simulink model "Simulacion_Completa_DET_M1"  (R2023a)
settings: Solver=VariableStepAuto  StartTime=0.0  StopTime=6062  RelTol=1e-3
undefined symbols (not defined in the file): Ion, Lithium
libraries: spsSeriesRLCBranchLib x15, spsIdealSwitchLib x11, slpidlib x3, spsCurrentMeasurementLib x2, spsIGBTDiodeLib x2, SignalEditorBlockLib x2, spsVoltageMeasurementLib x2, spsBatteryLib x1, spsBoostConverterLib x1, simulink x1, spsDiodeLib x1, eeGeneralControl x1
settings Model: SimulationMode=accelerator  Creator=javie  LastModifiedBy=javie
settings DebuggingCC: ParameterPrecisionLossMsg=none

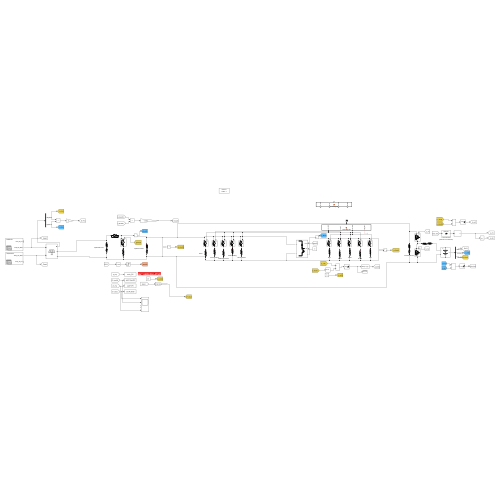
[thumbnail: Simulink's stored preview of the top-level diagram]
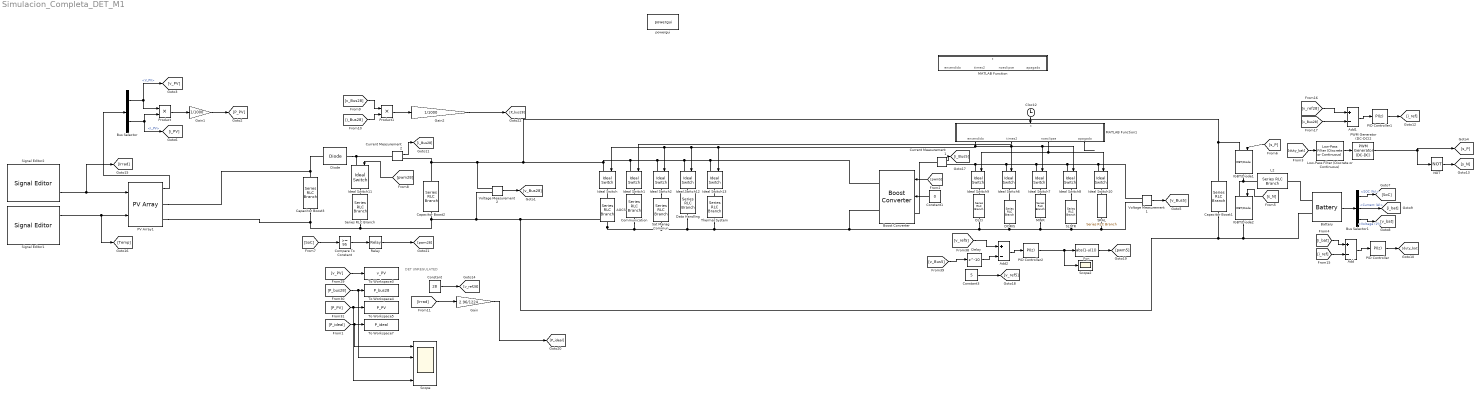
== system Simulacion_Completa_DET_M1 ==
  note: DET UNREGULATED
  AOCS : spsSeriesRLCBranchLib/Series RLC Branch  LConnTagsString=__new0  RConnTagsString=__new0  BranchType=R  Resistance=6.53  Inductance=1e-3  SetiL0=off  InitialCurrent=0  Capacitance=3300e-6  Setx0=off  InitialVoltage=0  Measurements=None
  Add : Sum  Inputs=+-
  Add1 : Sum  Inputs=+-
  Add2 : Sum  Inputs=+-
  Battery : spsBatteryLib/Battery  BatType=Lithium-Ion  ShowTempParam=off  ThermalPreset=no  ShowAgeParam=off  NomV=26  NomQ=60  SOC=60  Batt_Tr=1  PresetModel=on  MaxQ=60  MinV=19.5  FullV=30.2637  Dis_rate=26.087  R=0.0043333  Normal_OP=54.2609  expZone="[28.09      2.94783]"  current=[6.5 13 32.5]  Units=Time  Tci=20  NomT=20  T2=-30  MaxQ2=4.8  FullV2=7.1  Normal_OP2=5.655  expZone2="[6.58           1]"  Rca=0.6  ti=2000  Dp=0  Neq0=0  Tsim=1e6  Ta1=25  Qeol=5.4*0.9  Reol=0.013333*1.2  Char_age=[2.3478, 3]  Dis_age=[2.3478, 10]  N1=1500  N2=10500  N3=1000  N4=1400  Ta2=45  N5=950
  Boost Converter : spsBoostConverterLib/Boost Converter  ModelType=Average model (No rectifier mode)  Ron=1e-3  Rs=1e6  Cs=inf  Vforward=[0,0]  Ron_Diode=1e-3  Rs_Diode=1e6  Cs_Diode=inf  Vf_Diode=1e-3  Rs_CurrentSource=inf  Ron_ACsource=1e-3
      settings: LibrarySourceBlock=sps_lib/Power Electronics/Boost Converter
  Bus Selector : BusSelector  OutputSignals=V_PV,I_PV
  Bus Selector1 : BusSelector  OutputSignals=SOC (%),Current (A),Voltage (V)
  Capacitor Boost1 : spsSeriesRLCBranchLib/Series RLC Branch  LConnTagsString=__new0  RConnTagsString=__new0  BranchType=RC  Resistance=1e-4  Inductance=1e-3  SetiL0=off  InitialCurrent=0  Capacitance=1000e-6  Setx0=off  InitialVoltage=0  Measurements=None
  Capacitor Boost2 : spsSeriesRLCBranchLib/Series RLC Branch  LConnTagsString=__new0  RConnTagsString=__new0  BranchType=RC  Resistance=1e-4  Inductance=1e-3  SetiL0=off  InitialCurrent=0  Capacitance=1000e-6  Setx0=off  InitialVoltage=0  Measurements=None
  Capacitor Boost3 : spsSeriesRLCBranchLib/Series RLC Branch  LConnTagsString=__new0  RConnTagsString=__new0  BranchType=RC  Resistance=1e-4  Inductance=1e-3  SetiL0=off  InitialCurrent=0  Capacitance=1000e-6  Setx0=off  InitialVoltage=0  Measurements=None
  Clock2 : Clock
  Communication : spsSeriesRLCBranchLib/Series RLC Branch  LConnTagsString=__new0  RConnTagsString=__new0  BranchType=R  Resistance=5.23  Inductance=1e-3  SetiL0=off  InitialCurrent=0  Capacitance=3300e-6  Setx0=off  InitialVoltage=0  Measurements=None
  Compare To Constant : simulink/Logic and Bit Operations/Compare To Constant  relop=>=  const=95  OutDataTypeStr=boolean
  Constant : Constant  Value=28
  Constant1 : Constant  Value=0
  Constant3 : Constant  Value=5
  Current Measurement1 : spsCurrentMeasurementLib/Current Measurement  PhasorSimulation=off  OutputType=Complex  PSBequivalent=0
  Current Measurement2 : spsCurrentMeasurementLib/Current Measurement  PhasorSimulation=off  OutputType=Complex  PSBequivalent=0
  DORIS : spsSeriesRLCBranchLib/Series RLC Branch  LConnTagsString=__new0  RConnTagsString=__new0  BranchType=R  Resistance=1  Inductance=1e-3  SetiL0=off  InitialCurrent=0  Capacitance=3300e-6  Setx0=off  InitialVoltage=0  Measurements=None
  Data Handling : spsSeriesRLCBranchLib/Series RLC Branch  LConnTagsString=__new0  RConnTagsString=__new0  BranchType=R  Resistance=7.84  Inductance=1e-3  SetiL0=off  InitialCurrent=0  Capacitance=3300e-6  Setx0=off  InitialVoltage=0  Measurements=None
  Delay : Delay  DelayLength=10
  Diode : spsDiodeLib/Diode  Ron=0.001  Lon=0  Vf=0.8  IC=0  UseSnubber=0  Rs=500  Cs=250e-9  Measurements=off
  Fcn : Fcn  Expr=abs(1-u(1))
  Gain : Gain  Gain=2.96/1224  OutDataTypeStr=Inherit: Same as input
  Gain1 : Gain  Gain=1/1000
  Gain2 : Gain  Gain=1/1000
  IGBT/Diode1 : spsIGBTDiodeLib/IGBT//Diode  Ron=1e-3  Rs=1e5  Cs=inf  Measurements=off
  IGBT/Diode2 : spsIGBTDiodeLib/IGBT//Diode  Ron=1e-3  Rs=1e5  Cs=inf  Measurements=off
  Ideal Switch{,1..2,6..13} (11 alike) : spsIdealSwitchLib/Ideal Switch  Ron=0.001  Lon=0  IC=0  Rs=1e5  Cs=inf  Measurements=off
  L2 : spsSeriesRLCBranchLib/Series RLC Branch  LConnTagsString=__new0  RConnTagsString=__new0  BranchType=RL  Resistance=0.1  Inductance=0.5e-3  SetiL0=off  InitialCurrent=0  Capacitance=1e-6  Setx0=off  InitialVoltage=0  Measurements=None
  Low-Pass Filter (Discrete or Continuous) : eeGeneralControl/Low-Pass Filter (Discrete or Continuous)  K=1  T=1  B=inf  A=-inf  init_option=Inherited from block input  x0=0  Ts=-1
  MATLAB Function : MATLAB Function  TreatAsAtomicUnit=on
  MATLAB Function1 : MATLAB Function  TreatAsAtomicUnit=on
  MWR : spsSeriesRLCBranchLib/Series RLC Branch  LConnTagsString=__new0  RConnTagsString=__new0  BranchType=R  Resistance=0.74  Inductance=1e-3  SetiL0=off  InitialCurrent=0  Capacitance=3300e-6  Setx0=off  InitialVoltage=0  Measurements=None
  NOT : Logic  Operator=NOT  AllPortsSameDT=off  OutDataTypeStr=boolean
  OLCI : spsSeriesRLCBranchLib/Series RLC Branch  LConnTagsString=__new0  RConnTagsString=__new0  BranchType=R  Resistance=0.2  Inductance=1e-3  SetiL0=off  InitialCurrent=0  Capacitance=3300e-6  Setx0=off  InitialVoltage=0  Measurements=None
  PID Controller : slpidlib/PID Controller  Controller=PI  Form=Parallel  TimeDomain=Discrete-time  UseExternalTs=off  SampleTime=50e-6  IntegratorMethod=Forward Euler  FilterMethod=Forward Euler  ControllerParametersSource=internal  P=0.8  I=10  UseKiTs=off  D=0  N=100  UseFilter=on  TunerSelectOption=Frequency Response Based  InitialConditionSource=internal  InitialConditionForIntegrator=0  InitialConditionForFilter=0  DifferentiatorICPrevScaledInput=0  ExternalReset=none  TrackingMode=off  Kt=1  LimitOutput=on  SatLimitsSource=internal  UpperSaturationLimit=0.95  LowerSaturationLimit=0  LinearizeAsGain=on  AntiWindupMode=none  Kb=1  LimitIntegrator=off  UpperIntegratorSaturationLimit=inf  LowerIntegratorSaturationLimit=-inf  POutMin=[]  POutMax=[]  IOutMin=[]  IOutMax=[]  DOutMin=[]  DOutMax=[]  NOutMin=[]  NOutMax=[]  SumOutMin=[]  SumOutMax=[]  SaturationOutMin=[]  SaturationOutMax=[]  PParamMin=[]  PParamMax=[]  IParamMin=[]  IParamMax=[]  DParamMin=[]  DParamMax=[]  NParamMin=[]  NParamMax=[]  KbParamMin=[]  KbParamMax=[]  KtParamMin=[]  KtParamMax=[]  KbOutMin=[]  KbOutMax=[]  KtOutMin=[]  KtOutMax=[]  IntegratorOutMin=[]  IntegratorOutMax=[]  FilterOutMin=[]  FilterOutMax=[]  SumI1OutMin=[]  SumI1OutMax=[]  SumI2OutMin=[]  SumI2OutMax=[]  SumI3OutMin=[]  SumI3OutMax=[]  SumI4OutMin=[]  SumI4OutMax=[]  SumDOutMin=[]  SumDOutMax=[]  DifferentiatorOutMin=[]  DifferentiatorOutMax=[]  FilterDiffOutCoefMin=[]  FilterDiffOutCoefMax=[]  ReciprocalOutMin=[]  ReciprocalOutMax=[]  SumDenOutMin=[]  SumDenOutMax=[]  SumNumOutMin=[]  SumNumOutMax=[]  DivideOutMin=[]  DivideOutMax=[]  UdiffTsProdOutMin=[]  UdiffTsProdOutMax=[]  NTsProdOutMin=[]  NTsProdOutMax=[]  UintegralTsProdOutMin=[]  UintegralTsProdOutMax=[]  UngainTsProdOutMin=[]  UngainTsProdOutMax=[]  ClampingZeroOutDataTypeStr=Inherit: Inherit via back propagation  ClampingZeroOutMin=[]  ClampingZeroOutMax=[]  FilterDenConstantOutDataTypeStr=Inherit: Inherit via back propagation  FilterDenConstantOutMin=[]  FilterDenConstantOutMax=[]  PCopyOutDataTypeStr=Inherit: Inherit via back propagation  PCopyOutMin=[]  PCopyOutMax=[]  NCopyOutDataTypeStr=Inherit: Inherit via back propagation  NCopyOutMin=[]  NCopyOutMax=[]  IntegratorContinuousStateAttributes=''  IntegratorStateMustResolveToSignalObject=off  IntegratorRTWStateStorageClass=Auto  FilterContinuousStateAttributes=''  FilterStateMustResolveToSignalObject=off  FilterRTWStateStorageClass=Auto  ParallelPVariant=InternalParameters  IdealPVariant=Disabled  IVariant=InternalParameters  DVariant=Disabled  IntegratorVariant=Discrete  SatVariant=Enabled  AWVariant=Passthrough  PCopyVariant=Disabled  TRVariant=Disabled  FdbkBlocksVariant=Forward  IdealPFdbkVariant=Disabled  SatFdbkVariant=Disabled  DerivativeFilterVariant=Disabled  NVariant=Disabled  NCopyVariant=Disabled_SignalSpec  FilterICVariant=Disabled  IntegratorICVariant=InternalICs  ExternalResetVariant=Disabled  TRSumVariant=Passthrough  SumFdbkVariant=Disabled  SumVariant=Sum_PI  TsampFilterVariant=InternalTs  TsampNgainVariant=Passthrough  TsampIntegralVariant=Disabled_SignalSpec  ExternalSaturationOutDataTypeStr=Inherit: Same as second input
  PID Controller1 : slpidlib/PID Controller  Controller=PI  Form=Parallel  TimeDomain=Discrete-time  UseExternalTs=off  SampleTime=500e-6  IntegratorMethod=Forward Euler  FilterMethod=Forward Euler  ControllerParametersSource=internal  P=0.85  I=10  UseKiTs=off  D=0  N=100  UseFilter=on  TunerSelectOption=Transfer Function Based (PID Tuner App)  InitialConditionSource=internal  InitialConditionForIntegrator=0  InitialConditionForFilter=0  DifferentiatorICPrevScaledInput=0  ExternalReset=none  TrackingMode=off  Kt=1  LimitOutput=on  SatLimitsSource=internal  UpperSaturationLimit=40  LowerSaturationLimit=-40  LinearizeAsGain=on  AntiWindupMode=none  Kb=1  LimitIntegrator=off  UpperIntegratorSaturationLimit=inf  LowerIntegratorSaturationLimit=-inf  RndMeth=Zero  POutMin=[]  POutMax=[]  IOutMin=[]  IOutMax=[]  DOutMin=[]  DOutMax=[]  NOutMin=[]  NOutMax=[]  SumOutMin=[]  SumOutMax=[]  SaturationOutMin=[]  SaturationOutMax=[]  PParamMin=[]  PParamMax=[]  IParamMin=[]  IParamMax=[]  DParamMin=[]  DParamMax=[]  NParamMin=[]  NParamMax=[]  KbParamMin=[]  KbParamMax=[]  KtParamMin=[]  KtParamMax=[]  KbOutMin=[]  KbOutMax=[]  KtOutMin=[]  KtOutMax=[]  IntegratorOutMin=[]  IntegratorOutMax=[]  FilterOutMin=[]  FilterOutMax=[]  SumI1OutMin=[]  SumI1OutMax=[]  SumI2OutMin=[]  SumI2OutMax=[]  SumI3OutMin=[]  SumI3OutMax=[]  SumI4OutMin=[]  SumI4OutMax=[]  SumDOutMin=[]  SumDOutMax=[]  DifferentiatorOutMin=[]  DifferentiatorOutMax=[]  FilterDiffOutCoefMin=[]  FilterDiffOutCoefMax=[]  ReciprocalOutMin=[]  ReciprocalOutMax=[]  SumDenOutMin=[]  SumDenOutMax=[]  SumNumOutMin=[]  SumNumOutMax=[]  DivideOutMin=[]  DivideOutMax=[]  UdiffTsProdOutMin=[]  UdiffTsProdOutMax=[]  NTsProdOutMin=[]  NTsProdOutMax=[]  UintegralTsProdOutMin=[]  UintegralTsProdOutMax=[]  UngainTsProdOutMin=[]  UngainTsProdOutMax=[]  ClampingZeroOutDataTypeStr=Inherit: Inherit via back propagation  ClampingZeroOutMin=[]  ClampingZeroOutMax=[]  FilterDenConstantOutDataTypeStr=Inherit: Inherit via back propagation  FilterDenConstantOutMin=[]  FilterDenConstantOutMax=[]  PCopyOutDataTypeStr=Inherit: Inherit via back propagation  PCopyOutMin=[]  PCopyOutMax=[]  NCopyOutDataTypeStr=Inherit: Inherit via back propagation  NCopyOutMin=[]  NCopyOutMax=[]  IntegratorContinuousStateAttributes=''  IntegratorStateMustResolveToSignalObject=off  IntegratorRTWStateStorageClass=Auto  FilterContinuousStateAttributes=''  FilterStateMustResolveToSignalObject=off  FilterRTWStateStorageClass=Auto  ParallelPVariant=InternalParameters  IdealPVariant=Disabled  IVariant=InternalParameters  DVariant=Disabled  IntegratorVariant=Discrete  SatVariant=Enabled  AWVariant=Passthrough  PCopyVariant=Disabled  TRVariant=Disabled  FdbkBlocksVariant=Forward  IdealPFdbkVariant=Disabled  SatFdbkVariant=Disabled  DerivativeFilterVariant=Disabled  NVariant=Disabled  NCopyVariant=Disabled_SignalSpec  FilterICVariant=Disabled  IntegratorICVariant=InternalICs  ExternalResetVariant=Disabled  TRSumVariant=Passthrough  SumFdbkVariant=Disabled  SumVariant=Sum_PI  TsampFilterVariant=InternalTs  TsampNgainVariant=Passthrough  TsampIntegralVariant=Disabled_SignalSpec  ExternalSaturationOutDataTypeStr=Inherit: Same as second input
  PID Controller2 : slpidlib/PID Controller  Controller=PI  Form=Parallel  TimeDomain=Discrete-time  UseExternalTs=off  SampleTime=50e-6  IntegratorMethod=Forward Euler  FilterMethod=Forward Euler  ControllerParametersSource=internal  P=0.02  I=1  UseKiTs=off  D=0  N=100  UseFilter=on  TunerSelectOption=Frequency Response Based  InitialConditionSource=internal  InitialConditionForIntegrator=0  InitialConditionForFilter=0  DifferentiatorICPrevScaledInput=0  ExternalReset=none  TrackingMode=off  Kt=1  LimitOutput=on  SatLimitsSource=internal  UpperSaturationLimit=0.999  LowerSaturationLimit=0  LinearizeAsGain=off  AntiWindupMode=none  Kb=1  LimitIntegrator=off  UpperIntegratorSaturationLimit=inf  LowerIntegratorSaturationLimit=-inf  POutMin=[]  POutMax=[]  IOutMin=[]  IOutMax=[]  DOutMin=[]  DOutMax=[]  NOutMin=[]  NOutMax=[]  SumOutMin=[]  SumOutMax=[]  SaturationOutMin=[]  SaturationOutMax=[]  PParamMin=[]  PParamMax=[]  IParamMin=[]  IParamMax=[]  DParamMin=[]  DParamMax=[]  NParamMin=[]  NParamMax=[]  KbParamMin=[]  KbParamMax=[]  KtParamMin=[]  KtParamMax=[]  KbOutMin=[]  KbOutMax=[]  KtOutMin=[]  KtOutMax=[]  IntegratorOutMin=[]  IntegratorOutMax=[]  FilterOutMin=[]  FilterOutMax=[]  SumI1OutMin=[]  SumI1OutMax=[]  SumI2OutMin=[]  SumI2OutMax=[]  SumI3OutMin=[]  SumI3OutMax=[]  SumI4OutMin=[]  SumI4OutMax=[]  SumDOutMin=[]  SumDOutMax=[]  DifferentiatorOutMin=[]  DifferentiatorOutMax=[]  FilterDiffOutCoefMin=[]  FilterDiffOutCoefMax=[]  ReciprocalOutMin=[]  ReciprocalOutMax=[]  SumDenOutMin=[]  SumDenOutMax=[]  SumNumOutMin=[]  SumNumOutMax=[]  DivideOutMin=[]  DivideOutMax=[]  UdiffTsProdOutMin=[]  UdiffTsProdOutMax=[]  NTsProdOutMin=[]  NTsProdOutMax=[]  UintegralTsProdOutMin=[]  UintegralTsProdOutMax=[]  UngainTsProdOutMin=[]  UngainTsProdOutMax=[]  ClampingZeroOutDataTypeStr=Inherit: Inherit via back propagation  ClampingZeroOutMin=[]  ClampingZeroOutMax=[]  FilterDenConstantOutDataTypeStr=Inherit: Inherit via back propagation  FilterDenConstantOutMin=[]  FilterDenConstantOutMax=[]  PCopyOutDataTypeStr=Inherit: Inherit via back propagation  PCopyOutMin=[]  PCopyOutMax=[]  NCopyOutDataTypeStr=Inherit: Inherit via back propagation  NCopyOutMin=[]  NCopyOutMax=[]  IntegratorContinuousStateAttributes=''  IntegratorStateMustResolveToSignalObject=off  IntegratorRTWStateStorageClass=Auto  FilterContinuousStateAttributes=''  FilterStateMustResolveToSignalObject=off  FilterRTWStateStorageClass=Auto  ParallelPVariant=InternalParameters  IdealPVariant=Disabled  IVariant=InternalParameters  DVariant=Disabled  IntegratorVariant=Discrete  SatVariant=Enabled  AWVariant=Passthrough  PCopyVariant=Disabled  TRVariant=Disabled  FdbkBlocksVariant=Forward  IdealPFdbkVariant=Disabled  SatFdbkVariant=Disabled  DerivativeFilterVariant=Disabled  NVariant=Disabled  NCopyVariant=Disabled_SignalSpec  FilterICVariant=Disabled  IntegratorICVariant=InternalICs  ExternalResetVariant=Disabled  TRSumVariant=Passthrough  SumFdbkVariant=Disabled  SumVariant=Sum_PI  TsampFilterVariant=InternalTs  TsampNgainVariant=Passthrough  TsampIntegralVariant=Disabled_SignalSpec  ExternalSaturationOutDataTypeStr=Inherit: Same as second input
  PV Array1 : spsPVArrayLib/PV Array  Npar=7  Nser=2  PlotType=array @ 25 deg.C & specified irradiances  S_vec=[ 1200 1000 800 400 ]  Temp_C_vec="[ 45 25  ]"  ModuleName=Solartech Energy ASC-6P-48-180  PlotWhenSelected=off  Pm=180.0288  Ncell=48  Voc=29.2  Isc=8.48  Vm=22.56  Im=7.98  beta_Voc_pc=-0.36  alpha_Isc_pc=0.06  beta_Voc=-0.10512  alpha_Isc=0.005088  IL=8.5066  I0=2.8822e-10  nI=0.9824  Rsh=559.0814  Rs=0.40197  RobustModel=off  RobustCellTemperature=313.3991  BAL=on  Tc=1e-6  Tfilter=5e-5
  PWM Generator (DC-DC)2 : spsPWMGeneratorDCDCLib/PWM Generator (DC-DC)  Fsw=20000  Ts=1e-4
  Product : Product
  Product1 : Product
  Relay : Relay
  SLSTR : spsSeriesRLCBranchLib/Series RLC Branch  LConnTagsString=__new0  RConnTagsString=__new0  BranchType=R  Resistance=0.16  Inductance=1e-3  SetiL0=off  InitialCurrent=0  Capacitance=3300e-6  Setx0=off  InitialVoltage=0  Measurements=None
  SRAL : spsSeriesRLCBranchLib/Series RLC Branch  LConnTagsString=__new0  RConnTagsString=__new0  BranchType=R  Resistance=0.28  Inductance=1e-3  SetiL0=off  InitialCurrent=0  Capacitance=3300e-6  Setx0=off  InitialVoltage=0  Measurements=None
  Sat Manag Commun : spsSeriesRLCBranchLib/Series RLC Branch  LConnTagsString=__new0  RConnTagsString=__new0  BranchType=R  Resistance=6.03  Inductance=1e-3  SetiL0=off  InitialCurrent=0  Capacitance=3300e-6  Setx0=off  InitialVoltage=0  Measurements=None
  Scope : Scope  NumInputPorts=4
  Scope2 : Scope
  Series RLC Branch : spsSeriesRLCBranchLib/Series RLC Branch  LConnTagsString=__new0  RConnTagsString=__new0  BranchType=R  Resistance=1  Inductance=1e-3  SetiL0=off  InitialCurrent=0  Capacitance=1e-6  Setx0=off  InitialVoltage=0  Measurements=None
  Signal Editor1 : SignalEditorBlockLib/Signal Editor  FileName=Irradiancias_signal_6062.mat  ActiveScenario=Temperatura  ActiveSignal=Temp_50_6062  IsBus=off  OutputBusObjectStr=Bus: BusObject  SampleTime=0  Interpolate=off  ZeroCross=off  OutputAfterFinalValue=Setting to zero  Unit=inherit  PreserveSignalName=on  ApplySigPropsToAllScenarios=off
  Signal Editor2 : SignalEditorBlockLib/Signal Editor  FileName=Irradiancias_signal_6062.mat  ActiveScenario=Irradiancia  ActiveSignal=Irrad_50_10  IsBus=off  OutputBusObjectStr=Bus: BusObject  SampleTime=0  Interpolate=off  ZeroCross=off  OutputAfterFinalValue=Setting to zero  Unit=inherit  PreserveSignalName=on  ApplySigPropsToAllScenarios=off
  Thermal System : spsSeriesRLCBranchLib/Series RLC Branch  LConnTagsString=__new0  RConnTagsString=__new0  BranchType=R  Resistance=9.8  Inductance=1e-3  SetiL0=off  InitialCurrent=0  Capacitance=3300e-6  Setx0=off  InitialVoltage=0  Measurements=None
  To Workspace3 : ToWorkspace  VariableName=v_PV  SaveFormat=Structure With Time  SampleTime=-1
      settings: Decimation=10000
  To Workspace4 : ToWorkspace  VariableName=P_bus28  SaveFormat=Structure With Time  SampleTime=-1
      settings: Decimation=10000
  To Workspace5 : ToWorkspace  VariableName=P_PV  SaveFormat=Structure With Time  SampleTime=-1
      settings: Decimation=10000
  To Workspace7 : ToWorkspace  VariableName=P_ideal  SaveFormat=Structure With Time  SampleTime=-1
      settings: Decimation=10000
  Voltage Measurement1 : spsVoltageMeasurementLib/Voltage Measurement  PhasorSimulation=off  OutputType=Complex  PSBequivalent=0
  Voltage Measurement2 : spsVoltageMeasurementLib/Voltage Measurement  PhasorSimulation=off  OutputType=Complex  PSBequivalent=0
  powergui : sps_lib/powergui  Priority=1  SimulationMode=Discrete  SampleTime=1e-4  frequency=60  Iterations=50  frequencyindice=0  Pbase=100e6  ErrMax=1e-4  UnitsV=kV  UnitsW=MW  buscounter=0  FunctionMessages=off  echomessages=off  EnableUseOfTLC=off  CurrentSourceSwitches=off  DisableSnubberDevices=off  DisableRonSwitches=off  DisableVfSwitches=off  DisplayEquations=off  AutomaticDiscreteSolvers=off  SolverType=Tustin/Backward Euler (TBE)  Interpol=off  ExternalGateDelay=off  methode=off  Ts=100  x0status=blocks  SPID=on  SwTol=0  HookPort=off  NonlinearTolerance=1e-4  nMaxIteration=100  ContinueOnMaxIteration=off  RestoreLinks=warning  ResistiveCurrentMeasurement=off  Frange=[0:2:500]  Ylog=off  Xlog=on  ShowGrid=off  save=off  variable=ZData  structure=0  ZoomFFT=off  StartTime=0.0  cycles=1  DisplayStyle=1  fundamental=60  FreqAxis=off  MaxFrequency=1000  frequencyindicesteady=1  RmsSteady=1  display=off
  wires:
  [pwm28] -> Ideal Switch11/1
  Relay/1 -> [pwm28]
  [SoC] -> Compare To Constant/1
  Current Measurement2/1 -> [i_Bus28]
  Compare To Constant/1 -> Relay/1
  PV Array1/1 -> Bus Selector/1
  Gain1/1 -> [P_PV]
  Bus Selector/2 -> Product/2, [i_PV]  "<I_PV>"
  Bus Selector/1 -> Product/1, [v_PV]  "<V_PV>"
  Product/1 -> Gain1/1
  [P_ideal] -> Scope/1, To Workspace7/1
  [P_bus28] -> Scope/2, To Workspace4/1
  Constant/1 -> [v_ref28]
  [Irrad] -> Gain/1
  Gain/1 -> [P_ideal]
  [v_PV] -> To Workspace3/1
  [P_PV] -> Scope/4, To Workspace5/1
  [v_Bus28] -> Add1/2
  NOT/1 -> [s_N]
  [duty_bat] -> Low-Pass Filter (Discrete or Continuous)/1
  [s_P] -> IGBT/Diode1/1
  Add1/1 -> PID Controller1/1
  [i_bat] -> Add/1
  Bus Selector1/3 -> [v_bat]  "<Voltage (V)>"
  [v_ref28] -> Add1/1
  PWM Generator (DC-DC)2/1 -> [s_P], NOT/1
  [i_ref] -> Add/2
  PID Controller/1 -> [duty_bat]
  Battery/1 -> Bus Selector1/1
  Add/1 -> PID Controller/1
  Bus Selector1/1 -> [SoC]  "<SOC (%)>"
  [s_N] -> IGBT/Diode2/1
  Bus Selector1/2 -> [i_bat]  "<Current (A)>"
  Low-Pass Filter (Discrete or Continuous)/1 -> PWM Generator (DC-DC)2/1
  PID Controller1/1 -> [i_ref]
  Constant1/1 -> Boost Converter/2
  Add2/1 -> PID Controller2/1
  Fcn/1 -> [pwm5]
  Delay/1 -> Add2/2
  Current Measurement1/1 -> [i_Bus5]
  [v_Bus5] -> Delay/1
  Voltage Measurement1/1 -> [v_Bus5]
  Constant3/1 -> [v_ref5]
  MATLAB Function1/3(noeclipse) -> Ideal Switch10/1, Ideal Switch9/1
  [v_ref5] -> Add2/1
  PID Controller2/1 -> Scope2/1, Fcn/1
  Clock2/1 -> MATLAB Function1/1(t)
  [pwm5] -> Boost Converter/1
  MATLAB Function1/4(apagado) -> ?
  MATLAB Function1/1(encendido) -> Ideal Switch8/1, Ideal Switch7/1, Ideal Switch6/1, Ideal Switch/1, Ideal Switch2/1, Ideal Switch12/1, Ideal Switch13/1
  Signal Editor2/2 -> [Irrad], PV Array1/1
  Signal Editor1/1 -> [Temp], PV Array1/2
  MATLAB Function1/2(times2) -> Ideal Switch1/1
  Voltage Measurement2/1 -> [v_Bus28]
  Product1/1 -> Gain2/1
  Gain2/1 -> [P_bus28]
  [v_Bus28] -> Product1/1
  [i_Bus28] -> Product1/2
  connections:
  Diode/RConn1 -- Ideal Switch11/LConn1 -- Current Measurement2/LConn1
  Ideal Switch11/RConn1 -- Series RLC Branch/LConn1
  Diode/LConn1 -- PV Array1/RConn1 -- Capacitor Boost3/LConn1
  Capacitor Boost1/RConn1 -- Voltage Measurement2/LConn2 -- PV Array1/RConn2 -- Capacitor Boost3/RConn1 -- Series RLC Branch/RConn1 -- Capacitor Boost2/RConn1 -- Communication/RConn1 -- Sat Manag Commun/RConn1 -- Data Handling/RConn1 -- Boost Converter/RConn2 -- OLCI/RConn1 -- DORIS/RConn1 -- MWR/RConn1 -- SLSTR/RConn1 -- SRAL/RConn1 -- Voltage Measurement1/LConn2 -- Thermal System/RConn1 -- AOCS/RConn1 -- Battery/LConn2 -- IGBT/Diode2/RConn1
  L2/LConn1 -- IGBT/Diode1/RConn1 -- IGBT/Diode2/LConn1
  Ideal Switch/LConn1 -- Capacitor Boost1/LConn1 -- IGBT/Diode1/LConn1 -- Voltage Measurement2/LConn1 -- Current Measurement2/RConn1 -- Capacitor Boost2/LConn1 -- Ideal Switch1/LConn1 -- Boost Converter/RConn1 -- Ideal Switch13/LConn1 -- Ideal Switch12/LConn1 -- Ideal Switch2/LConn1
  Battery/LConn1 -- L2/RConn1
  Current Measurement1/RConn1 -- Ideal Switch9/LConn1 -- Ideal Switch6/LConn1 -- Ideal Switch7/LConn1 -- Voltage Measurement1/LConn1 -- Ideal Switch10/LConn1 -- Ideal Switch8/LConn1
  OLCI/LConn1 -- Ideal Switch9/RConn1
  Ideal Switch10/RConn1 -- SRAL/LConn1
  AOCS/LConn1 -- Ideal Switch/RConn1
  DORIS/LConn1 -- Ideal Switch6/RConn1
  Thermal System/LConn1 -- Ideal Switch13/RConn1
  Boost Converter/LConn1 -- Current Measurement1/LConn1
  MWR/LConn1 -- Ideal Switch7/RConn1
  Data Handling/LConn1 -- Ideal Switch12/RConn1
  Ideal Switch1/RConn1 -- Communication/LConn1
  Ideal Switch2/RConn1 -- Sat Manag Commun/LConn1
  Ideal Switch8/RConn1 -- SLSTR/LConn1

== matlab function Simulacion_Completa_DET_M1/MATLAB Function ==
  data: t input; encendido output; times2 output; noeclipse output; apagado output
function [encendido, times2, noeclipse, apagado] = controlSignals(t)
    % Inicializa las señales en 0
    encendido = 1;
    times2 = 0;
    noeclipse = 1;
    apagado = 0;
    
    
    % Activa times2 entre 10 y 11 segundos
    if (t >= 3 && t < 3.1)
        times2 = 1;
    end

    if (t >= 9.2 && t < 9.3)
        times2 = 1;
    end
    % Activa la señal3 entre 10 y 11 segundos
    if (t >= 3.6 && t < 8.2)
        noeclipse = 0;
    end
end

== matlab function Simulacion_Completa_DET_M1/MATLAB Function1 ==
  data: t input; encendido output; times2 output; noeclipse output; apagado output
function [encendido, times2, noeclipse, apagado] = controlSignals(t)
    % Inicializa las señales en 0
    encendido = 1;
    times2 = 0;
    noeclipse = 1;
    apagado = 0;
    
    
    % Activa times2 entre 10 y 11 segundos
    if (t >= 300 && t < 330)
        times2 = 1;
    end

    if (t >= 6000 && t < 6030)
        times2 = 1;
    end
    % Activa la señal3 entre 10 y 11 segundos
    if (t >= 2020 && t < 5050)
        noeclipse = 0;
    end
end
